simulink model "singleMassMPCcontinus2017"  (R2017a)
settings: Solver=VariableStepAuto  StartTime=0.0  StopTime=16  RelTol=1e-3
libraries: simulink x1
settings Model: Creator=daoist  LastModifiedBy=daoist
settings DataIOCC: ReturnWorkspaceOutputs=on
settings DebuggingCC: SFMachineParentedDataDiag=error
settings SFSimCC: SimUseLocalCustomCode=on
settings RTWCC: RTWUseLocalCustomCode=on

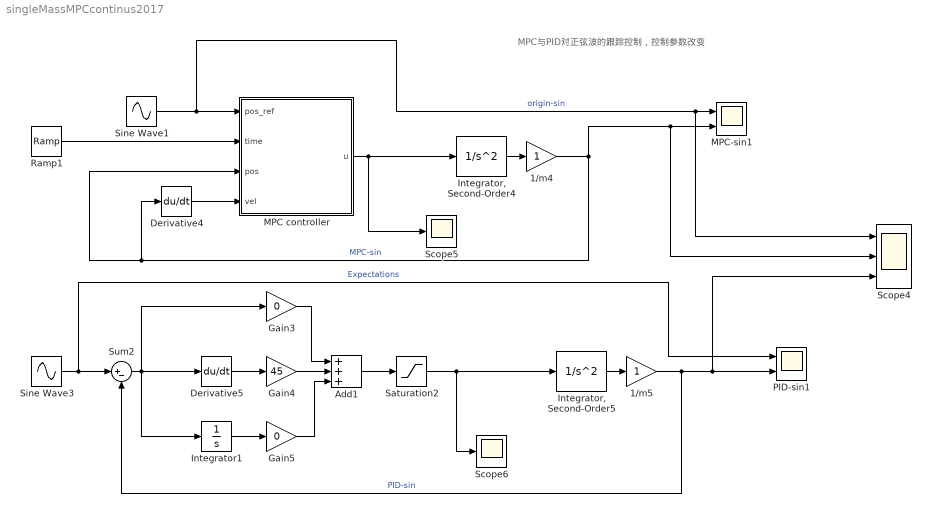
== system singleMassMPCcontinus2017 ==
  note: MPC与PID对正弦波的跟踪控制，控制参数改变
  1/m4 : Gain
  1/m5 : Gain
  Add1 : Sum  Inputs=+++
  Derivative4 : Derivative
  Derivative5 : Derivative
  Gain3 : Gain  Gain=0
  Gain4 : Gain  Gain=45
  Gain5 : Gain  Gain=0
  "Integrator, Second-Order4" : SecondOrderIntegrator  ShowOutput=x
  "Integrator, Second-Order5" : SecondOrderIntegrator  ShowOutput=x
  Integrator1 : Integrator
  MPC controller : MATLAB Function  TreatAsAtomicUnit=on
  MPC-sin1 : Scope  NumInputPorts=2
  PID-sin1 : Scope  NumInputPorts=2
  Ramp1 : simulink/Sources/Ramp  slope=1  start=0  X0=0
  Saturation2 : Saturate  UpperLimit=100  LowerLimit=-100
  Scope4 : Scope  NumInputPorts=3
  Scope5 : Scope
  Scope6 : Scope
  Sine Wave1 : Sin  Frequency=pi  SampleTime=0
  Sine Wave3 : Sin  Frequency=pi  SampleTime=0
  Sum2 : Sum  Inputs=|+-
  wires:
  Gain4/1 -> Add1/2
  MPC controller/1(u) -> "Integrator, Second-Order4"/1, Scope5/1
  Gain5/1 -> Add1/3
  Sum2/1 -> Integrator1/1, Derivative5/1, Gain3/1
  1/m4/1 -> Scope4/2, MPC-sin1/2, MPC controller/3(pos), Derivative4/1  "MPC-sin"
  Ramp1/1 -> MPC controller/2(time)
  Sine Wave1/1 -> Scope4/1, MPC-sin1/1, MPC controller/1(pos_ref)  "origin-sin"
  "Integrator, Second-Order5"/1 -> 1/m5/1
  Integrator1/1 -> Gain5/1
  1/m5/1 -> Scope4/3, PID-sin1/2, Sum2/2  "PID-sin"
  Sine Wave3/1 -> Sum2/1, PID-sin1/1  "Expectations"
  Derivative5/1 -> Gain4/1
  "Integrator, Second-Order4"/1 -> 1/m4/1
  Gain3/1 -> Add1/1
  Derivative4/1 -> MPC controller/4(vel)
  Add1/1 -> Saturation2/1
  Saturation2/1 -> "Integrator, Second-Order5"/1, Scope6/1

== matlab function singleMassMPCcontinus2017/MPC controller ==
  data: pos_ref input size=1; time input; pos input size=1; vel input size=1; u output size=1
function u = MPCcontroller(pos_ref, time, pos, vel)
%参数设置
m    = 1.05;          %滑块质量,增加了5%作为建模误差
T    = 0.1;           %控制周期100ms
p    = 40;            %控制时域（预测时域）
Q    = 10*eye(2*p);   %累计误差权重
W    = 0.0001*eye(p); %控制输出权重
% umax = 100;          
umax = 100 * ones(p); %控制量限制，即最大的力
Rk   = zeros(2*p,1);  %参考值序列
timeseris = time:T:time+T*(p-1);
Rk(1:2:end) = sin(pi()*(timeseris+0.1 ))*1.05;    
Rk(2:2:end) = pi()*cos(pi()*(timeseris+0.1))*1.05;    %参考速度
%构建中间变量
xk    = [pos;vel];    %xk
A_    = [1 T;0 1];    %离散化预测模型参数A
B_    = [0;T/m];      %离散化预测模型参数B
B_    = [T^2/m/2;T/m]; 
psi   = zeros(2*p,2); %psi
for i=1:1:p
    psi(i*2-1:i*2,1:2)=A_^i;
end
theta = zeros(2*p,p); %theta
for i=1:1:p
    for j=1:1:i
        theta(i*2-1:i*2,j)=A_^(i-j)*B_;
    end
end
E = psi*xk-Rk;            %E
H = 2*(theta'*Q*theta+W); %H
f = (2*E'*Q*theta)';      %f
%优化求解
coder.extrinsic('quadprog');
Uk=quadprog(H,f,[],[],[],[],-umax,umax);
%返回控制量序列第一个值
u = 0.0;                %显示指定u的类型
u = Uk(1);
